simulink model "Part1"  (R2024b)
settings: Solver=VariableStepAuto  StartTime=0.0  StopTime=10.0  RelTol=1e-3
settings Model: Creator=baley  LastModifiedBy=baley

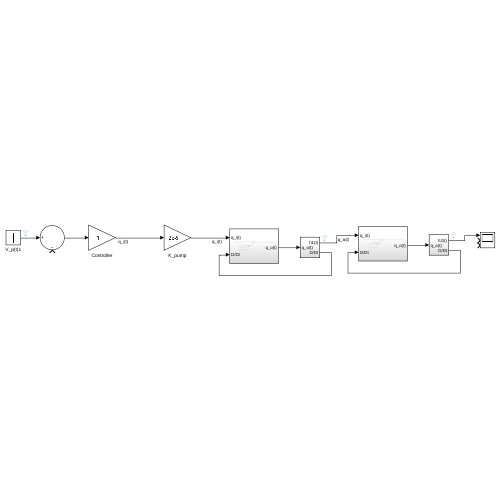
[thumbnail: Simulink's stored preview of the top-level diagram]
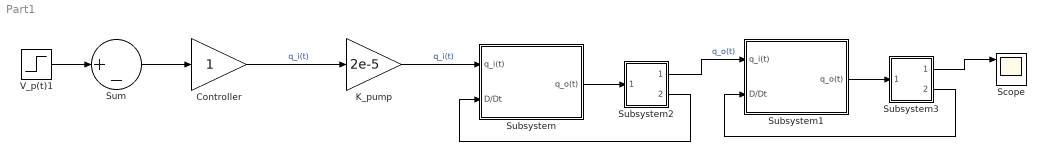
== system Part1 ==
  Controller : Gain
  K_pump : Gain  Gain=2e-5
  Scope : Scope  NumInputPorts=3
  Subsystem : Subsystem
  Subsystem1 : Subsystem
  Subsystem2 : Subsystem
  Subsystem3 : Subsystem
  Sum : Sum  Inputs=|+-
  V_p(t)1 : Step  Before=1  After=2  SampleTime=0
  wires:
  K_pump/1 -> Subsystem/1(q_i(t))  "q_i(t)"
  Subsystem/1(q_o(t)) -> Subsystem2/1(q_o(t))
  Subsystem2/2(D/Dt) -> Subsystem/2(D/Dt)
  Subsystem2/1(h1(t)) -> Subsystem1/1(q_i(t))  "q_o(t)"
  Subsystem1/1(q_o(t)) -> Subsystem3/1(q_o(t))
  Subsystem3/2(D/Dt) -> Subsystem1/2(D/Dt)
  Controller/1 -> K_pump/1  "q_i(t)"
  V_p(t)1/1 -> Sum/1
  Sum/1 -> Controller/1
  Subsystem3/1(h2(t)) -> Scope/1

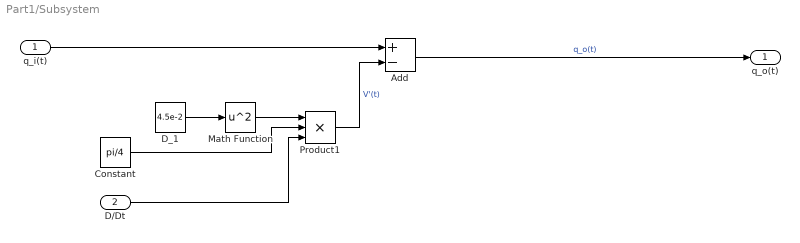
== system Part1/Subsystem ==
  q_i(t) : Inport
  D/Dt : Inport  Port=2
  Add : Sum  Inputs=+-
  Constant : Constant  Value=pi/4
  D_1 : Constant  Value=4.5e-2
  Math Function : Math  Operator=square
  Product1 : Product  Inputs=3
  q_o(t) : Outport
  wires:
  Constant/1 -> Product1/2
  D_1/1 -> Math Function/1
  Add/1 -> q_o(t)/1  "q_o(t)"
  Math Function/1 -> Product1/1
  q_i(t)/1 -> Add/1
  Product1/1 -> Add/2  "V'(t)"
  D/Dt/1 -> Product1/3

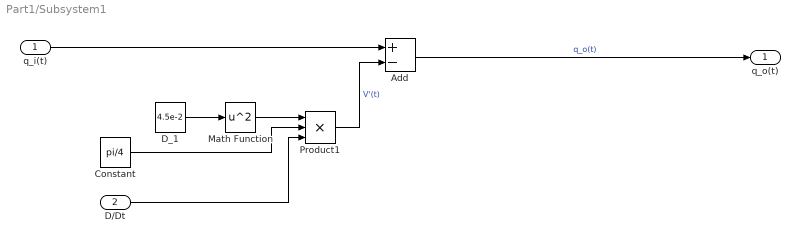
== system Part1/Subsystem1 ==
  q_i(t) : Inport
  D/Dt : Inport  Port=2
  Add : Sum  Inputs=+-
  Constant : Constant  Value=pi/4
  D_1 : Constant  Value=4.5e-2
  Math Function : Math  Operator=square
  Product1 : Product  Inputs=3
  q_o(t) : Outport
  wires:
  Constant/1 -> Product1/2
  D_1/1 -> Math Function/1
  Add/1 -> q_o(t)/1  "q_o(t)"
  Math Function/1 -> Product1/1
  q_i(t)/1 -> Add/1
  Product1/1 -> Add/2  "V'(t)"
  D/Dt/1 -> Product1/3

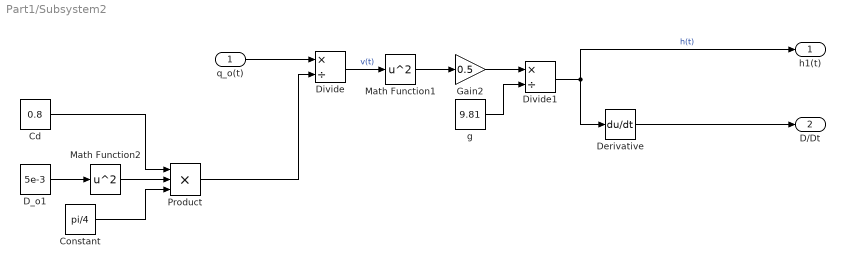
== system Part1/Subsystem2 ==
  q_o(t) : Inport
  Cd : Constant  Value=0.8
  Constant : Constant  Value=pi/4
  D_o1 : Constant  Value=5e-3
  Derivative : Derivative
  Divide : Product  Inputs=*/
  Divide1 : Product  Inputs=*/
  Gain2 : Gain  Gain=0.5
  Math Function1 : Math  Operator=square
  Math Function2 : Math  Operator=square
  Product : Product  Inputs=3
  g : Constant  Value=9.81
  h1(t) : Outport
  D/Dt : Outport  Port=2
  wires:
  q_o(t)/1 -> Divide/1
  Math Function2/1 -> Product/2
  Gain2/1 -> Divide1/1
  Derivative/1 -> D/Dt/1
  Constant/1 -> Product/3
  Product/1 -> Divide/2
  Divide1/1 -> h1(t)/1, Derivative/1  "h(t)"
  Math Function1/1 -> Gain2/1
  Cd/1 -> Product/1
  Divide/1 -> Math Function1/1  "v(t)"
  g/1 -> Divide1/2
  D_o1/1 -> Math Function2/1

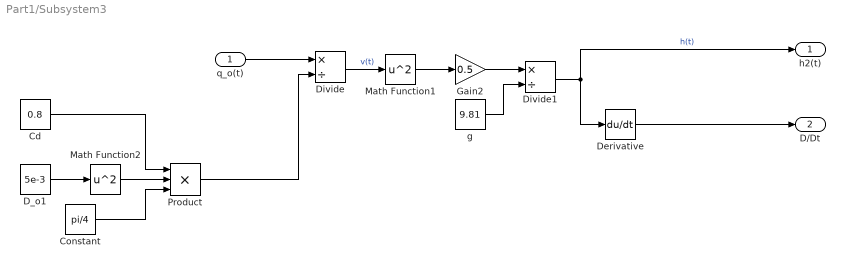
== system Part1/Subsystem3 ==
  q_o(t) : Inport
  Cd : Constant  Value=0.8
  Constant : Constant  Value=pi/4
  D_o1 : Constant  Value=5e-3
  Derivative : Derivative
  Divide : Product  Inputs=*/
  Divide1 : Product  Inputs=*/
  Gain2 : Gain  Gain=0.5
  Math Function1 : Math  Operator=square
  Math Function2 : Math  Operator=square
  Product : Product  Inputs=3
  g : Constant  Value=9.81
  h2(t) : Outport
  D/Dt : Outport  Port=2
  wires:
  q_o(t)/1 -> Divide/1
  Math Function2/1 -> Product/2
  Gain2/1 -> Divide1/1
  Derivative/1 -> D/Dt/1
  Constant/1 -> Product/3
  Product/1 -> Divide/2
  Divide1/1 -> h2(t)/1, Derivative/1  "h(t)"
  Math Function1/1 -> Gain2/1
  Cd/1 -> Product/1
  Divide/1 -> Math Function1/1  "v(t)"
  g/1 -> Divide1/2
  D_o1/1 -> Math Function2/1
